simulink model "PE_V2_0"  (R2020b)
settings: Solver=VariableStepAuto  StartTime=0.0  StopTime=10.0  RelTol=1e-3
undefined symbols (not defined in the file): ZERO
libraries: hdlsllib x35, simulink x28, visionhdlutilities x12
(part 1 of 3)
settings Model: Creator=Xiao  LastModifiedBy=Xiao

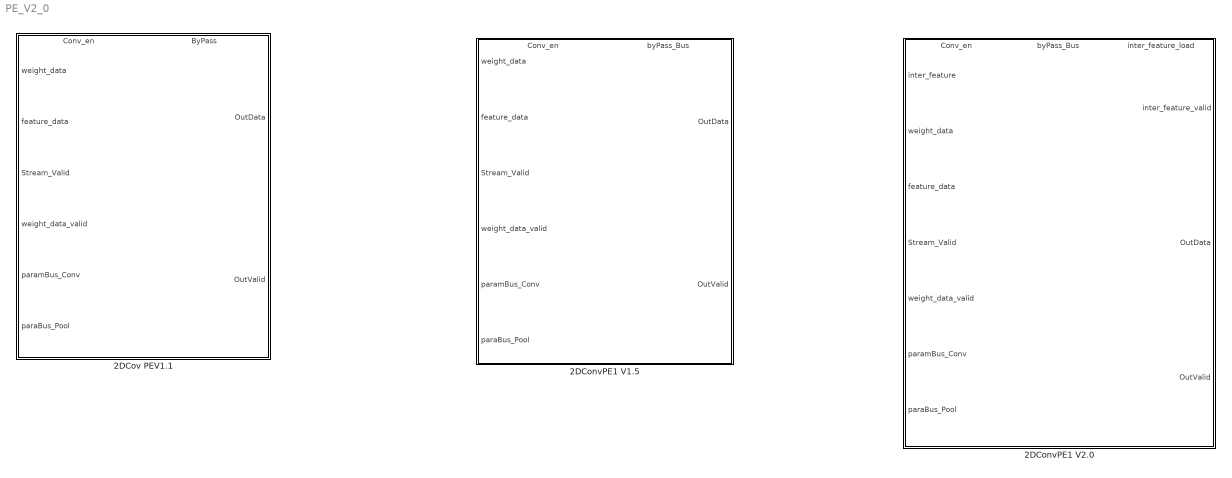
== system PE_V2_0 ==
  2DConvPE1 V1.5 : Subsystem
      settings: PortSchema="{\"entries\":[{\"content\":{\"sides\":[{\"content\":{\"connectorIds\":[\"In1\",\"In2\",\"In3\",\"In4\",\"In5\",\"In6\"]},\"type\":\"ConnectorPlacement.EquallySpacedRectSide\",\"uuid\":\"72a132f7-3e47-4ef1-8d79-baadbeb84817\"},{\"content\":{\"connectorIds\":[\"Out1\",\"Out2\"],\"side\":\"RIGHT\"},\"type\":\"ConnectorPlacement.EquallySpacedRectSide\",\"uuid\":\"2df9bf31-2175-4d97-aafa-a0227f37f2af\"},{\"content\":{\"connectorIds\":[\"In7\",\"In8\"],\"side\":\"TOP\"},\"type\":\"ConnectorPlacement.EquallySpacedRectSide\",\"uuid\":\"1b8495b8-ab7c-42d9-b044-413e20debbac\"},{\"content\":{\"connectorIds\":[],\"side\":\"BOTTOM\"},\"type\":\"ConnectorPlacement.EquallySpacedRectSide\",\"uuid\":\"e68361ac-7f7b-4816-948a-9cecfdd8f729\"},{\"content\":{\"connectorIds\":[],\"side\":\"HIDDEN\"},\"type\":\"ConnectorPlacement.EquallySpacedRectSide\",\"uuid\":\"818be012-dd2c-438f-8537-4d3d95a16bb4\"}]},\"type\":\"ConnectorPlacement.EquallySpacedConnector\",\"uuid\":\"cbadf64c-68f0-4765-b1bf-d60756169ff2\"}],\"packageUris\":[\"http://schema.mathworks.com/mf0/Connector/R2020b\"],\"version\":\"1.0\"}"
  2DConvPE1 V2.0 : Subsystem
      settings: PortSchema="{\"entries\":[{\"content\":{\"sides\":[{\"content\":{\"connectorIds\":[\"In1\",\"In2\",\"In3\",\"In4\",\"In5\",\"In6\",\"In7\"]},\"type\":\"ConnectorPlacement.EquallySpacedRectSide\",\"uuid\":\"72a132f7-3e47-4ef1-8d79-baadbeb84817\"},{\"content\":{\"connectorIds\":[\"Out1\",\"Out2\",\"Out3\"],\"side\":\"RIGHT\"},\"type\":\"ConnectorPlacement.EquallySpacedRectSide\",\"uuid\":\"2df9bf31-2175-4d97-aafa-a0227f37f2af\"},{\"content\":{\"connectorIds\":[\"In8\",\"In9\",\"In10\"],\"side\":\"TOP\"},\"type\":\"ConnectorPlacement.EquallySpacedRectSide\",\"uuid\":\"1b8495b8-ab7c-42d9-b044-413e20debbac\"},{\"content\":{\"connectorIds\":[],\"side\":\"BOTTOM\"},\"type\":\"ConnectorPlacement.EquallySpacedRectSide\",\"uuid\":\"e68361ac-7f7b-4816-948a-9cecfdd8f729\"},{\"content\":{\"connectorIds\":[],\"side\":\"HIDDEN\"},\"type\":\"ConnectorPlacement.EquallySpacedRectSide\",\"uuid\":\"818be012-dd2c-438f-8537-4d3d95a16bb4\"}]},\"type\":\"ConnectorPlacement.EquallySpacedConnector\",\"uuid\":\"cbadf64c-68f0-4765-b1bf-d60756169ff2\"}],\"packageUris\":[\"http://schema.mathworks.com/mf0/Connector/R2020b\"],\"version\":\"1.0\"}"
  2DCov PEV1.1 : Subsystem
      settings: PortSchema="{\"entries\":[{\"content\":{\"sides\":[{\"content\":{\"connectorIds\":[\"In1\",\"In2\",\"In3\",\"In4\",\"In5\",\"In6\"]},\"type\":\"ConnectorPlacement.EquallySpacedRectSide\",\"uuid\":\"72a132f7-3e47-4ef1-8d79-baadbeb84817\"},{\"content\":{\"connectorIds\":[\"Out1\",\"Out2\"],\"side\":\"RIGHT\"},\"type\":\"ConnectorPlacement.EquallySpacedRectSide\",\"uuid\":\"2df9bf31-2175-4d97-aafa-a0227f37f2af\"},{\"content\":{\"connectorIds\":[\"In7\",\"In8\"],\"side\":\"TOP\"},\"type\":\"ConnectorPlacement.EquallySpacedRectSide\",\"uuid\":\"1b8495b8-ab7c-42d9-b044-413e20debbac\"},{\"content\":{\"connectorIds\":[],\"side\":\"BOTTOM\"},\"type\":\"ConnectorPlacement.EquallySpacedRectSide\",\"uuid\":\"e68361ac-7f7b-4816-948a-9cecfdd8f729\"},{\"content\":{\"connectorIds\":[],\"side\":\"HIDDEN\"},\"type\":\"ConnectorPlacement.EquallySpacedRectSide\",\"uuid\":\"818be012-dd2c-438f-8537-4d3d95a16bb4\"}]},\"type\":\"ConnectorPlacement.EquallySpacedConnector\",\"uuid\":\"cbadf64c-68f0-4765-b1bf-d60756169ff2\"}],\"packageUris\":[\"http://schema.mathworks.com/mf0/Connector/R2020b\"],\"version\":\"1.0\"}"

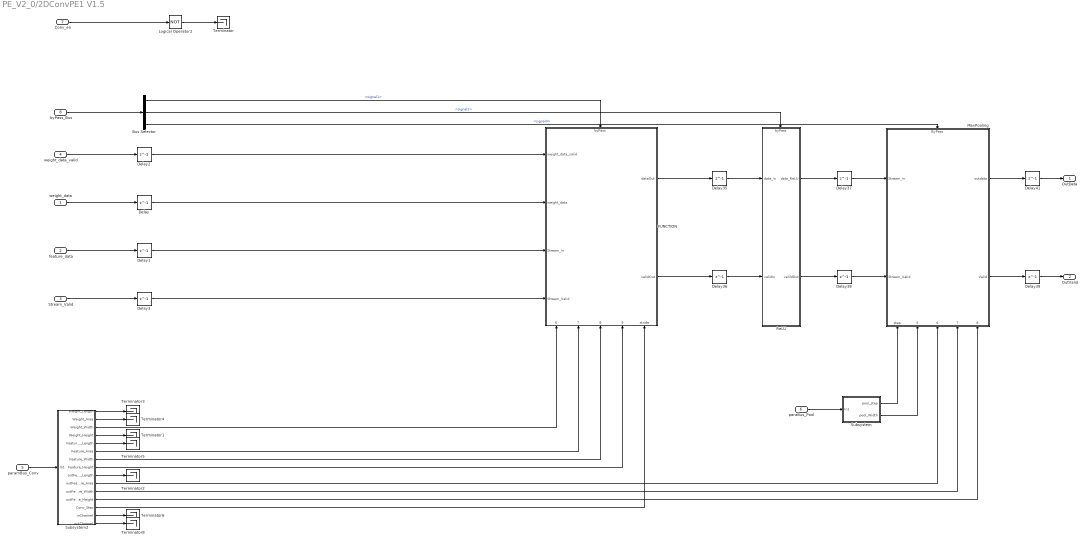
== system PE_V2_0/2DConvPE1 V1.5 ==
  weight_data : Inport
  feature_data : Inport  Port=2
  Stream_Valid : Inport  Port=3
  weight_data_valid : Inport  Port=4
  paramBus_Conv : Inport  Port=5
  paraBus_Pool : Inport  Port=6
  Conv_en : Inport  Port=7
  byPass_Bus : Inport  Port=8
  Bus Selector : BusSelector  OutputSignals=signal1,signal2,signal3
  Delay{,1..3,35..39,41} (10 alike) : Delay  DelayLength=1
  FUNCTION : Subsystem
      settings: PortSchema="{\"entries\":[{\"content\":{\"sides\":[{\"content\":{\"connectorIds\":[\"In1\",\"In2\",\"In3\",\"In4\"]},\"type\":\"ConnectorPlacement.EquallySpacedRectSide\",\"uuid\":\"bed083cc-10ce-4f46-a724-2c2c82e71793\"},{\"content\":{\"connectorIds\":[\"Out1\",\"Out2\"],\"side\":\"RIGHT\"},\"type\":\"ConnectorPlacement.EquallySpacedRectSide\",\"uuid\":\"c0d53dd0-88dc-4789-a28b-52aa625e6829\"},{\"content\":{\"connectorIds\":[\"In5\"],\"side\":\"TOP\"},\"type\":\"ConnectorPlacement.EquallySpacedRectSide\",\"uuid\":\"1fc99caf-d887-47fd-8f7a-576d1660cb35\"},{\"content\":{\"connectorIds\":[\"In6\",\"In7\",\"In8\",\"In9\",\"In10\"],\"side\":\"BOTTOM\"},\"type\":\"ConnectorPlacement.EquallySpacedRectSide\",\"uuid\":\"c33a9856-e25e-4d20-97d3-ef7dd12e1c8d\"},{\"content\":{\"connectorIds\":[],\"side\":\"HIDDEN\"},\"type\":\"ConnectorPlacement.EquallySpacedRectSide\",\"uuid\":\"c30f7557-1904-42a6-8652-95c43c5090df\"}]},\"type\":\"ConnectorPlacement.EquallySpacedConnector\",\"uuid\":\"8e0cb07a-0a7c-4542-b766-635afc6aa2db\"}],\"packageUris\":[\"http://schema.mathworks.com/mf0/Connector/R2020b\"],\"version\":\"1.0\"}"
  Logical Operator2 : Logic  Operator=NOT  AllPortsSameDT=off  OutDataTypeStr=boolean
  MaxPooling : Subsystem
      settings: PortSchema="{\"entries\":[{\"content\":{\"sides\":[{\"content\":{\"connectorIds\":[\"In1\",\"In2\"]},\"type\":\"ConnectorPlacement.EquallySpacedRectSide\",\"uuid\":\"8f082555-10a5-4426-9c6d-30ad9c9edc83\"},{\"content\":{\"connectorIds\":[\"Out1\",\"Out2\"],\"side\":\"RIGHT\"},\"type\":\"ConnectorPlacement.EquallySpacedRectSide\",\"uuid\":\"2f08e48d-98a7-49ef-9240-49e9a92f7835\"},{\"content\":{\"connectorIds\":[\"In3\"],\"side\":\"TOP\"},\"type\":\"ConnectorPlacement.EquallySpacedRectSide\",\"uuid\":\"9c785374-bdb9-47d6-a84c-95016a7dac24\"},{\"content\":{\"connectorIds\":[\"In4\",\"In5\",\"In6\",\"In7\",\"In8\"],\"side\":\"BOTTOM\"},\"type\":\"ConnectorPlacement.EquallySpacedRectSide\",\"uuid\":\"81220b33-16bc-4efc-91f7-9bf9738f949c\"},{\"content\":{\"connectorIds\":[],\"side\":\"HIDDEN\"},\"type\":\"ConnectorPlacement.EquallySpacedRectSide\",\"uuid\":\"99d22b10-fe8c-4c64-8a09-c433657226d7\"}]},\"type\":\"ConnectorPlacement.EquallySpacedConnector\",\"uuid\":\"f09d9050-86eb-4a30-82a2-eebdb84e68d3\"}],\"packageUris\":[\"http://schema.mathworks.com/mf0/Connector/R2020b\"],\"version\":\"1.0\"}"
  ReLU : Subsystem
      settings: PortSchema="{\"entries\":[{\"content\":{\"sides\":[{\"content\":{\"connectorIds\":[\"In1\",\"In2\"]},\"type\":\"ConnectorPlacement.EquallySpacedRectSide\",\"uuid\":\"abc19905-3b44-4985-b45b-942e5eaa1386\"},{\"content\":{\"connectorIds\":[\"Out1\",\"Out2\"],\"side\":\"RIGHT\"},\"type\":\"ConnectorPlacement.EquallySpacedRectSide\",\"uuid\":\"b0a86706-72e5-448b-9f1b-a0967f50aac9\"},{\"content\":{\"connectorIds\":[\"In3\"],\"side\":\"TOP\"},\"type\":\"ConnectorPlacement.EquallySpacedRectSide\",\"uuid\":\"df5d57b0-52e5-439f-8896-63a90ec5378c\"},{\"content\":{\"connectorIds\":[],\"side\":\"HIDDEN\"},\"type\":\"ConnectorPlacement.EquallySpacedRectSide\",\"uuid\":\"493b8843-365c-4ea1-b4d2-a52d72a7a785\"}]},\"type\":\"ConnectorPlacement.EquallySpacedConnector\",\"uuid\":\"755c5668-4a5f-4120-9a22-1155c417e52d\"}],\"packageUris\":[\"http://schema.mathworks.com/mf0/Connector/R2020b\"],\"version\":\"1.0\"}"
  Subsystem : Subsystem
  Subsystem2 : Subsystem
  Terminator{,1..6,8} (8 alike) : Terminator
  OutData : Outport
  OutValid : Outport  Port=2
  wires:
  Conv_en/1 -> Logical Operator2/1
  Logical Operator2/1 -> Terminator/1
  Delay35/1 -> ReLU/1(data_in)
  ReLU/1(data_ReLU) -> Delay37/1
  MaxPooling/1(outdata) -> Delay41/1
  MaxPooling/2(Valid) -> Delay39/1
  paraBus_Pool/1 -> Subsystem/1(In1)
  Subsystem/1(pool_step) -> MaxPooling/4(step)
  Subsystem/2(pool_Width) -> MaxPooling/5(Window_Width)
  Subsystem2/11(outFeature_Width) -> MaxPooling/7(Feature_Width)
  Subsystem2/10(outFeature_Area) -> MaxPooling/6(Feature_Area)
  Subsystem2/12(outFeature_Height) -> MaxPooling/8(Feature_Height)
  paramBus_Conv/1 -> Subsystem2/1(In1)
  Subsystem2/14(inChannel) -> Terminator6/1
  Subsystem2/4(Weight_Height) -> Terminator1/1
  Subsystem2/9(outFeature_Length) -> Terminator2/1
  Subsystem2/1(Weight_Length) -> Terminator3/1
  Subsystem2/2(Weight_Area) -> Terminator4/1
  Subsystem2/5(Feature_Length) -> Terminator5/1
  Subsystem2/15(outChannel) -> Terminator8/1
  ReLU/2(valildOut) -> Delay38/1
  weight_data/1 -> Delay/1
  weight_data_valid/1 -> Delay2/1
  feature_data/1 -> Delay1/1
  Stream_Valid/1 -> Delay3/1
  Delay36/1 -> ReLU/2(validIn)
  Delay37/1 -> MaxPooling/1(Stream_In)
  Delay38/1 -> MaxPooling/2(Stream_Valid)
  Delay41/1 -> OutData/1
  Delay39/1 -> OutValid/1
  byPass_Bus/1 -> Bus Selector/1
  Bus Selector/3 -> MaxPooling/3(ByPass)  "<signal3>"
  Bus Selector/2 -> ReLU/3(byPass)  "<signal2>"
  Delay2/1 -> FUNCTION/1(weight_data_valid)
  Delay/1 -> FUNCTION/2(weight_data)
  Delay1/1 -> FUNCTION/3(Stream_In)
  Delay3/1 -> FUNCTION/4(Stream_Valid)
  Subsystem2/3(Weight_Width) -> FUNCTION/6(Weight_Width)
  Subsystem2/6(Feature_Area) -> FUNCTION/7(Feature_Area)
  Subsystem2/7(Feature_Width) -> FUNCTION/8(Feature_Width)
  Subsystem2/8(Feature_Height) -> FUNCTION/9(Feature_Height)
  Subsystem2/13(Conv_Step) -> FUNCTION/10(stride)
  FUNCTION/1(dataOut) -> Delay35/1
  FUNCTION/2(validOut) -> Delay36/1
  Bus Selector/1 -> FUNCTION/5(byPass)  "<signal1>"

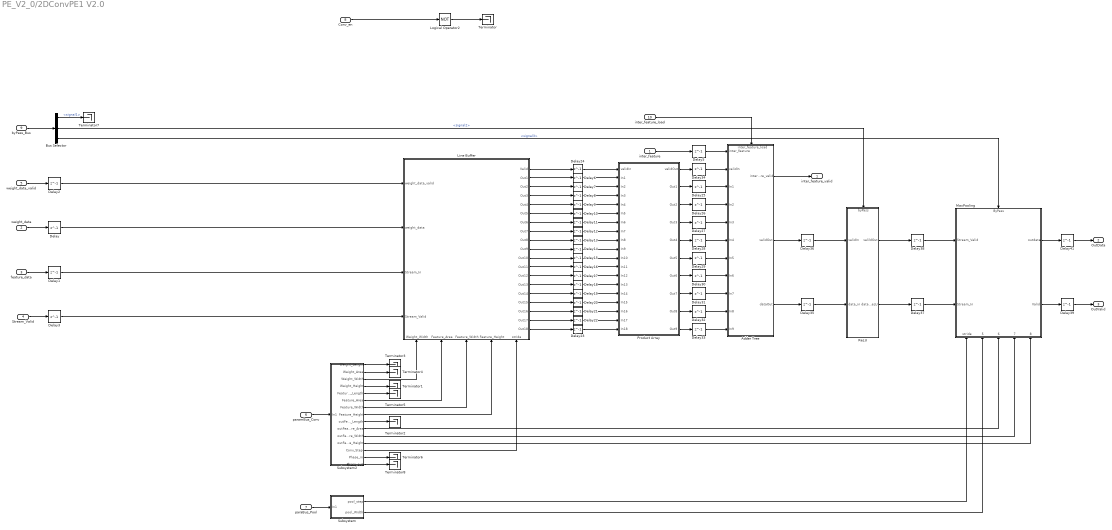
== system PE_V2_0/2DConvPE1 V2.0 ==
  inter_feature : Inport
  weight_data : Inport  Port=2
  feature_data : Inport  Port=3
  Stream_Valid : Inport  Port=4
  weight_data_valid : Inport  Port=5
  paramBus_Conv : Inport  Port=6
  paraBus_Pool : Inport  Port=7
  Conv_en : Inport  Port=8
  byPass_Bus : Inport  Port=9
  inter_feature_load : Inport  Port=10
  Adder Tree : Subsystem
      settings: PortSchema="{\"entries\":[{\"content\":{\"sides\":[{\"content\":{\"connectorIds\":[\"In1\",\"In2\",\"In3\",\"In4\",\"In5\",\"In6\",\"In7\",\"In8\",\"In9\",\"In10\",\"In11\"]},\"type\":\"ConnectorPlacement.EquallySpacedRectSide\",\"uuid\":\"a2770fc8-c2bb-4f97-8127-9a4f9dcf3825\"},{\"content\":{\"connectorIds\":[\"Out1\",\"Out2\",\"Out3\"],\"side\":\"RIGHT\"},\"type\":\"ConnectorPlacement.EquallySpacedRectSide\",\"uuid\":\"e7824c27-562b-441e-9955-8b5c243004da\"},{\"content\":{\"connectorIds\":[\"In12\"],\"side\":\"TOP\"},\"type\":\"ConnectorPlacement.EquallySpacedRectSide\",\"uuid\":\"ac1c8bec-6be4-4eb3-bc0e-7b7fb253fd27\"},{\"content\":{\"connectorIds\":[],\"side\":\"HIDDEN\"},\"type\":\"ConnectorPlacement.EquallySpacedRectSide\",\"uuid\":\"83260308-97e6-439f-9ad4-eb453db87a9c\"}]},\"type\":\"ConnectorPlacement.EquallySpacedConnector\",\"uuid\":\"e705b5d7-213e-4592-b0c5-9ab5c3365200\"}],\"packageUris\":[\"http://schema.mathworks.com/mf0/Connector/R2020b\"],\"version\":\"1.0\"}"
  Bus Selector : BusSelector  OutputSignals=signal1,signal2,signal3
  Delay{,1..3,5..39,41} (40 alike) : Delay  DelayLength=1
  Line Buffer : Subsystem
      settings: PortSchema="{\"entries\":[{\"content\":{\"sides\":[{\"content\":{\"connectorIds\":[\"In1\",\"In2\",\"In3\",\"In4\"]},\"type\":\"ConnectorPlacement.EquallySpacedRectSide\",\"uuid\":\"29b80ed8-848a-41c0-b6e7-f177bb4434f3\"},{\"content\":{\"connectorIds\":[\"Out1\",\"Out2\",\"Out3\",\"Out4\",\"Out5\",\"Out6\",\"Out7\",\"Out8\",\"Out9\",\"Out10\",\"Out11\",\"Out12\",\"Out13\",\"Out14\",\"Out15\",\"Out16\",\"Out17\",\"Out18\",\"Out19\"],\"side\":\"RIGHT\"},\"type\":\"ConnectorPlacement.EquallySpacedRectSide\",\"uuid\":\"adaf16a8-ce9f-43de-8b43-956a28d6fbef\"},{\"content\":{\"connectorIds\":[],\"side\":\"TOP\"},\"type\":\"ConnectorPlacement.EquallySpacedRectSide\",\"uuid\":\"106fd3d1-022d-44b8-9392-934ec241d21c\"},{\"content\":{\"connectorIds\":[\"In5\",\"In6\",\"In7\",\"In8\",\"In9\"],\"side\":\"BOTTOM\"},\"type\":\"ConnectorPlacement.EquallySpacedRectSide\",\"uuid\":\"8507e472-68b8-4fe5-bb7c-5a7beeecdd12\"},{\"content\":{\"connectorIds\":[],\"side\":\"HIDDEN\"},\"type\":\"ConnectorPlacement.EquallySpacedRectSide\",\"uuid\":\"f49b73e9-0f9f-4778-9ce1-2ad9bbb71891\"}]},\"type\":\"ConnectorPlacement.EquallySpacedConnector\",\"uuid\":\"21a60f11-360c-44f0-bdd6-bae5bf125dc3\"}],\"packageUris\":[\"http://schema.mathworks.com/mf0/Connector/R2020b\"],\"version\":\"1.0\"}"
  Logical Operator2 : Logic  Operator=NOT  AllPortsSameDT=off  OutDataTypeStr=boolean
  MaxPooling : Subsystem
      settings: PortSchema="{\"entries\":[{\"content\":{\"sides\":[{\"content\":{\"connectorIds\":[\"In1\",\"In2\"]},\"type\":\"ConnectorPlacement.EquallySpacedRectSide\",\"uuid\":\"8f082555-10a5-4426-9c6d-30ad9c9edc83\"},{\"content\":{\"connectorIds\":[\"Out1\",\"Out2\"],\"side\":\"RIGHT\"},\"type\":\"ConnectorPlacement.EquallySpacedRectSide\",\"uuid\":\"2f08e48d-98a7-49ef-9240-49e9a92f7835\"},{\"content\":{\"connectorIds\":[\"In3\"],\"side\":\"TOP\"},\"type\":\"ConnectorPlacement.EquallySpacedRectSide\",\"uuid\":\"9c785374-bdb9-47d6-a84c-95016a7dac24\"},{\"content\":{\"connectorIds\":[\"In4\",\"In5\",\"In6\",\"In7\",\"In8\"],\"side\":\"BOTTOM\"},\"type\":\"ConnectorPlacement.EquallySpacedRectSide\",\"uuid\":\"81220b33-16bc-4efc-91f7-9bf9738f949c\"},{\"content\":{\"connectorIds\":[],\"side\":\"HIDDEN\"},\"type\":\"ConnectorPlacement.EquallySpacedRectSide\",\"uuid\":\"99d22b10-fe8c-4c64-8a09-c433657226d7\"}]},\"type\":\"ConnectorPlacement.EquallySpacedConnector\",\"uuid\":\"f09d9050-86eb-4a30-82a2-eebdb84e68d3\"}],\"packageUris\":[\"http://schema.mathworks.com/mf0/Connector/R2020b\"],\"version\":\"1.0\"}"
  Product Array : Subsystem
  ReLU : Subsystem
      settings: PortSchema="{\"entries\":[{\"content\":{\"sides\":[{\"content\":{\"connectorIds\":[\"In1\",\"In2\"]},\"type\":\"ConnectorPlacement.EquallySpacedRectSide\",\"uuid\":\"abc19905-3b44-4985-b45b-942e5eaa1386\"},{\"content\":{\"connectorIds\":[\"Out1\",\"Out2\"],\"side\":\"RIGHT\"},\"type\":\"ConnectorPlacement.EquallySpacedRectSide\",\"uuid\":\"b0a86706-72e5-448b-9f1b-a0967f50aac9\"},{\"content\":{\"connectorIds\":[\"In3\"],\"side\":\"TOP\"},\"type\":\"ConnectorPlacement.EquallySpacedRectSide\",\"uuid\":\"df5d57b0-52e5-439f-8896-63a90ec5378c\"},{\"content\":{\"connectorIds\":[],\"side\":\"HIDDEN\"},\"type\":\"ConnectorPlacement.EquallySpacedRectSide\",\"uuid\":\"493b8843-365c-4ea1-b4d2-a52d72a7a785\"}]},\"type\":\"ConnectorPlacement.EquallySpacedConnector\",\"uuid\":\"755c5668-4a5f-4120-9a22-1155c417e52d\"}],\"packageUris\":[\"http://schema.mathworks.com/mf0/Connector/R2020b\"],\"version\":\"1.0\"}"
  Subsystem : Subsystem
  Subsystem2 : Subsystem
  Terminator{,1..8} (9 alike) : Terminator
  inter_feature_valid : Outport
  OutData : Outport  Port=2
  OutValid : Outport  Port=3
  wires:
  Conv_en/1 -> Logical Operator2/1
  Logical Operator2/1 -> Terminator/1
  Delay35/1 -> ReLU/2(data_in)
  ReLU/2(data_ReLU) -> Delay37/1
  MaxPooling/1(outdata) -> Delay41/1
  MaxPooling/2(Valid) -> Delay39/1
  paraBus_Pool/1 -> Subsystem/1(In1)
  Subsystem/1(pool_step) -> MaxPooling/4(stride)
  Subsystem/2(pool_Width) -> MaxPooling/5(Window_Width)
  Subsystem2/11(outFeature_Width) -> MaxPooling/7(Feature_Width)
  Subsystem2/10(outFeature_Area) -> MaxPooling/6(Feature_Area)
  Subsystem2/12(outFeature_Height) -> MaxPooling/8(Feature_Height)
  paramBus_Conv/1 -> Subsystem2/1(In1)
  Subsystem2/14(Phase_in) -> Terminator6/1
  Subsystem2/4(Weight_Height) -> Terminator1/1
  Subsystem2/9(outFeature_Length) -> Terminator2/1
  Subsystem2/1(Weight_Length) -> Terminator3/1
  Subsystem2/2(Weight_Area) -> Terminator4/1
  Subsystem2/5(Feature_Length) -> Terminator5/1
  Subsystem2/15(Phase_out) -> Terminator8/1
  ReLU/1(valildOut) -> Delay38/1
  weight_data/1 -> Delay/1
  weight_data_valid/1 -> Delay2/1
  feature_data/1 -> Delay1/1
  Stream_Valid/1 -> Delay3/1
  Delay36/1 -> ReLU/1(validIn)
  Delay37/1 -> MaxPooling/2(Stream_In)
  Delay38/1 -> MaxPooling/1(Stream_Valid)
  Delay41/1 -> OutData/1
  Delay39/1 -> OutValid/1
  byPass_Bus/1 -> Bus Selector/1
  Bus Selector/3 -> MaxPooling/3(ByPass)  "<signal3>"
  Bus Selector/2 -> ReLU/3(byPass)  "<signal2>"
  Adder Tree/3(dataOut) -> Delay35/1
  Adder Tree/2(validOut) -> Delay36/1
  Delay3/1 -> Line Buffer/4(Stream_Valid)
  Delay1/1 -> Line Buffer/3(Stream_In)
  Delay/1 -> Line Buffer/2(weight_data)
  Delay2/1 -> Line Buffer/1(weight_data_valid)
  Subsystem2/8(Feature_Height) -> Line Buffer/8(Feature_Height)
  Subsystem2/6(Feature_Area) -> Line Buffer/6(Feature_Area)
  Subsystem2/3(Weight_Width) -> Line Buffer/5(Weight_Width)
  Line Buffer/6(Out5) -> Delay10/1
  Line Buffer/5(Out4) -> Delay9/1
  Line Buffer/13(Out12) -> Delay17/1
  Line Buffer/3(Out2) -> Delay7/1
  Line Buffer/9(Out8) -> Delay13/1
  Line Buffer/8(Out7) -> Delay12/1
  Delay25/1 -> Adder Tree/3(In1)
  Line Buffer/7(Out6) -> Delay11/1
  Delay27/1 -> Adder Tree/5(In3)
  Delay29/1 -> Adder Tree/7(In5)
  Line Buffer/17(Out16) -> Delay21/1
  Delay26/1 -> Adder Tree/4(In2)
  Product Array/2(Out1) -> Delay25/1
  Delay33/1 -> Adder Tree/11(In9)
  Product Array/1(validOut) -> Delay34/1
  Product Array/9(Out8) -> Delay32/1
  Line Buffer/11(Out10) -> Delay15/1
  Delay30/1 -> Adder Tree/8(In6)
  Line Buffer/15(Out14) -> Delay19/1
  Delay31/1 -> Adder Tree/9(In7)
  Product Array/3(Out2) -> Delay26/1
  Product Array/5(Out4) -> Delay28/1
  Delay32/1 -> Adder Tree/10(In8)
  Product Array/6(Out5) -> Delay29/1
  Product Array/4(Out3) -> Delay27/1
  Line Buffer/4(Out3) -> Delay8/1
  Product Array/10(Out9) -> Delay33/1
  Delay24/1 -> Product Array/1(validIn)
  Delay28/1 -> Adder Tree/6(In4)
  Delay23/1 -> Product Array/19(In18)
  Subsystem2/13(Conv_Step) -> Line Buffer/9(stride)
  Product Array/8(Out7) -> Delay31/1
  Delay16/1 -> Product Array/12(In11)
  Delay19/1 -> Product Array/15(In14)
  Delay21/1 -> Product Array/17(In16)
  Delay17/1 -> Product Array/13(In12)
  Delay8/1 -> Product Array/4(In3)
  Line Buffer/12(Out11) -> Delay16/1
  Delay22/1 -> Product Array/18(In17)
  Delay14/1 -> Product Array/10(In9)
  Line Buffer/19(Out18) -> Delay23/1
  Line Buffer/2(Out1) -> Delay6/1
  Delay15/1 -> Product Array/11(In10)
  Line Buffer/16(Out15) -> Delay20/1
  Delay34/1 -> Adder Tree/2(validIn)
  Delay11/1 -> Product Array/7(In6)
  Line Buffer/18(Out17) -> Delay22/1
  Delay13/1 -> Product Array/9(In8)
  Line Buffer/14(Out13) -> Delay18/1
  Delay9/1 -> Product Array/5(In4)
  Delay20/1 -> Product Array/16(In15)
  Delay18/1 -> Product Array/14(In13)
  Subsystem2/7(Feature_Width) -> Line Buffer/7(Feature_Width)
  Delay12/1 -> Product Array/8(In7)
  Delay10/1 -> Product Array/6(In5)
  Delay6/1 -> Product Array/2(In1)
  Line Buffer/1(Valid) -> Delay24/1
  Product Array/7(Out6) -> Delay30/1
  Delay7/1 -> Product Array/3(In2)
  Line Buffer/10(Out9) -> Delay14/1
  Bus Selector/1 -> Terminator7/1  "<signal1>"
  inter_feature/1 -> Delay5/1
  Delay5/1 -> Adder Tree/1(inter_feature)
  inter_feature_load/1 -> Adder Tree/12(inter_feature_load)
  Adder Tree/1(inter_feature_valid) -> inter_feature_valid/1

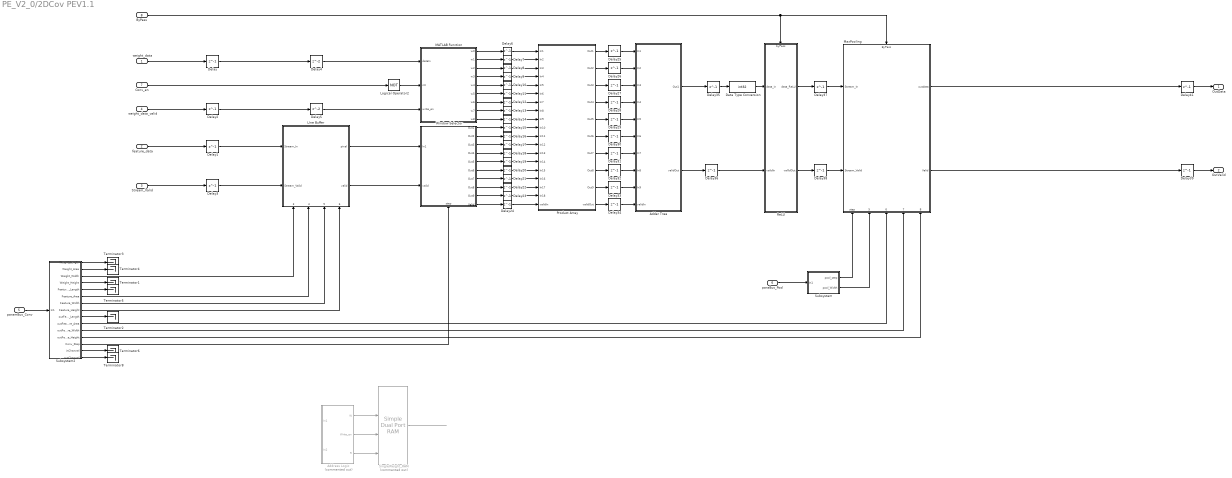
== system PE_V2_0/2DCov PEV1.1 ==
  weight_data : Inport
  feature_data : Inport  Port=2
  Stream_Valid : Inport  Port=3
  weight_data_valid : Inport  Port=4
  paramBus_Conv : Inport  Port=5
  paraBus_Pool : Inport  Port=6
  Conv_en : Inport  Port=7
  ByPass : Inport  Port=8
  Adder Tree : Subsystem
  Address Logic : Subsystem  Commented=on
  Data Type Conversion : DataTypeConversion  OutDataTypeStr=int32
  Delay{,1..3,6..39,41} (39 alike) : Delay  DelayLength=1
  Delay4 : Delay
  Delay5 : Delay
  LIne Buffer : Subsystem
      settings: PortSchema="{\"entries\":[{\"content\":{\"sides\":[{\"content\":{\"connectorIds\":[\"In1\",\"In2\"]},\"type\":\"ConnectorPlacement.EquallySpacedRectSide\",\"uuid\":\"a250c848-7a40-462c-bfcf-0ff48046d99d\"},{\"content\":{\"connectorIds\":[\"Out1\",\"Out2\"],\"side\":\"RIGHT\"},\"type\":\"ConnectorPlacement.EquallySpacedRectSide\",\"uuid\":\"81aecf2d-6bfb-4d40-80c7-cfb89c921406\"},{\"content\":{\"connectorIds\":[],\"side\":\"TOP\"},\"type\":\"ConnectorPlacement.EquallySpacedRectSide\",\"uuid\":\"288ccc7a-b219-4526-a408-3d8b1082f4b0\"},{\"content\":{\"connectorIds\":[\"In3\",\"In4\",\"In5\",\"In6\"],\"side\":\"BOTTOM\"},\"type\":\"ConnectorPlacement.EquallySpacedRectSide\",\"uuid\":\"5d9529f5-ee70-4412-83ca-b280a2219284\"},{\"content\":{\"connectorIds\":[],\"side\":\"HIDDEN\"},\"type\":\"ConnectorPlacement.EquallySpacedRectSide\",\"uuid\":\"3d06d450-49b0-49ba-a273-690d97c3e8e1\"}]},\"type\":\"ConnectorPlacement.EquallySpacedConnector\",\"uuid\":\"b82e05d1-4695-4e04-9663-17698b30471b\"}],\"packageUris\":[\"http://schema.mathworks.com/mf0/Connector/R2020b\"],\"version\":\"1.0\"}"
  Logical Operator2 : Logic  Operator=NOT  AllPortsSameDT=off  OutDataTypeStr=boolean
  MATLAB Function : MATLAB Function  TreatAsAtomicUnit=on
  MaxPooling : Subsystem
      settings: PortSchema="{\"entries\":[{\"content\":{\"sides\":[{\"content\":{\"connectorIds\":[\"In1\",\"In2\"]},\"type\":\"ConnectorPlacement.EquallySpacedRectSide\",\"uuid\":\"8f082555-10a5-4426-9c6d-30ad9c9edc83\"},{\"content\":{\"connectorIds\":[\"Out1\",\"Out2\"],\"side\":\"RIGHT\"},\"type\":\"ConnectorPlacement.EquallySpacedRectSide\",\"uuid\":\"2f08e48d-98a7-49ef-9240-49e9a92f7835\"},{\"content\":{\"connectorIds\":[\"In3\"],\"side\":\"TOP\"},\"type\":\"ConnectorPlacement.EquallySpacedRectSide\",\"uuid\":\"9c785374-bdb9-47d6-a84c-95016a7dac24\"},{\"content\":{\"connectorIds\":[\"In4\",\"In5\",\"In6\",\"In7\",\"In8\"],\"side\":\"BOTTOM\"},\"type\":\"ConnectorPlacement.EquallySpacedRectSide\",\"uuid\":\"81220b33-16bc-4efc-91f7-9bf9738f949c\"},{\"content\":{\"connectorIds\":[],\"side\":\"HIDDEN\"},\"type\":\"ConnectorPlacement.EquallySpacedRectSide\",\"uuid\":\"99d22b10-fe8c-4c64-8a09-c433657226d7\"}]},\"type\":\"ConnectorPlacement.EquallySpacedConnector\",\"uuid\":\"f09d9050-86eb-4a30-82a2-eebdb84e68d3\"}],\"packageUris\":[\"http://schema.mathworks.com/mf0/Connector/R2020b\"],\"version\":\"1.0\"}"
  Product Array : Subsystem
  ReLU : Subsystem
      settings: PortSchema="{\"entries\":[{\"content\":{\"sides\":[{\"content\":{\"connectorIds\":[\"In1\",\"In2\"]},\"type\":\"ConnectorPlacement.EquallySpacedRectSide\",\"uuid\":\"abc19905-3b44-4985-b45b-942e5eaa1386\"},{\"content\":{\"connectorIds\":[\"Out1\",\"Out2\"],\"side\":\"RIGHT\"},\"type\":\"ConnectorPlacement.EquallySpacedRectSide\",\"uuid\":\"b0a86706-72e5-448b-9f1b-a0967f50aac9\"},{\"content\":{\"connectorIds\":[\"In3\"],\"side\":\"TOP\"},\"type\":\"ConnectorPlacement.EquallySpacedRectSide\",\"uuid\":\"df5d57b0-52e5-439f-8896-63a90ec5378c\"},{\"content\":{\"connectorIds\":[],\"side\":\"HIDDEN\"},\"type\":\"ConnectorPlacement.EquallySpacedRectSide\",\"uuid\":\"493b8843-365c-4ea1-b4d2-a52d72a7a785\"}]},\"type\":\"ConnectorPlacement.EquallySpacedConnector\",\"uuid\":\"755c5668-4a5f-4120-9a22-1155c417e52d\"}],\"packageUris\":[\"http://schema.mathworks.com/mf0/Connector/R2020b\"],\"version\":\"1.0\"}"
  SingleWeight_RAM : hdlsllib/HDL RAMs/Simple Dual Port RAM  Commented=on  ram_size=13
      settings: SourceProductName=HDL Coder
  Subsystem : Subsystem
  Subsystem2 : Subsystem
  Terminator{1..6,8} (7 alike) : Terminator
  Window Selector : Subsystem
      settings: PortSchema="{\"entries\":[{\"content\":{\"sides\":[{\"content\":{\"connectorIds\":[\"In1\",\"In2\"]},\"type\":\"ConnectorPlacement.EquallySpacedRectSide\",\"uuid\":\"2f98ee57-d732-418e-86bd-7acbaf2524e0\"},{\"content\":{\"connectorIds\":[\"Out1\",\"Out2\",\"Out3\",\"Out4\",\"Out5\",\"Out6\",\"Out7\",\"Out8\",\"Out9\",\"Out10\"],\"side\":\"RIGHT\"},\"type\":\"ConnectorPlacement.EquallySpacedRectSide\",\"uuid\":\"287ad403-178f-48f1-9791-2ccad363e9c6\"},{\"content\":{\"connectorIds\":[],\"side\":\"TOP\"},\"type\":\"ConnectorPlacement.EquallySpacedRectSide\",\"uuid\":\"a860ecae-5cde-45ef-a487-fdb4fb7390aa\"},{\"content\":{\"connectorIds\":[\"In3\"],\"side\":\"BOTTOM\"},\"type\":\"ConnectorPlacement.EquallySpacedRectSide\",\"uuid\":\"925435f5-0fb8-4a67-9f76-fe99b5b92634\"},{\"content\":{\"connectorIds\":[],\"side\":\"HIDDEN\"},\"type\":\"ConnectorPlacement.EquallySpacedRectSide\",\"uuid\":\"e6f3edac-a41a-4276-8ae6-cd8be9b02af9\"}]},\"type\":\"ConnectorPlacement.EquallySpacedConnector\",\"uuid\":\"0e32a9d0-da82-46c8-ab50-9de41c4380a9\"}],\"packageUris\":[\"http://schema.mathworks.com/mf0/Connector/R2020b\"],\"version\":\"1.0\"}"
  OutData : Outport
  OutValid : Outport  Port=2
  wires:
  Delay/1 -> Delay4/1
  Address Logic/1(W) -> SingleWeight_RAM/2
  Address Logic/2(Write_en) -> SingleWeight_RAM/3
  Address Logic/3(R) -> SingleWeight_RAM/4
  SingleWeight_RAM/1 -> ?
  Conv_en/1 -> Logical Operator2/1
  Delay2/1 -> Delay5/1
  Logical Operator2/1 -> MATLAB Function/2(rst)
  Adder Tree/1(Out1) -> Delay35/1
  Data Type Conversion/1 -> ReLU/1(data_in)
  ReLU/1(data_ReLU) -> Delay37/1
  ByPass/1 -> MaxPooling/3(ByPass), ReLU/3(byPass)
  MaxPooling/1(outdata) -> Delay41/1
  MaxPooling/2(Valid) -> Delay39/1
  paraBus_Pool/1 -> Subsystem/1(In1)
  Subsystem/1(pool_step) -> MaxPooling/4(step)
  Subsystem/2(pool_Width) -> MaxPooling/5(Window_Width)
  Subsystem2/11(outFeature_Width) -> MaxPooling/7(Feature_Width)
  Subsystem2/10(outFeature_Area) -> MaxPooling/6(Feature_Area)
  Subsystem2/12(outFeature_Height) -> MaxPooling/8(Feature_Height)
  paramBus_Conv/1 -> Subsystem2/1(In1)
  Subsystem2/14(inChannel) -> Terminator6/1
  Subsystem2/4(Weight_Height) -> Terminator1/1
  Subsystem2/9(outFeature_Length) -> Terminator2/1
  Subsystem2/13(Conv_Step) -> Window Selector/3(step)
  Subsystem2/1(Weight_Length) -> Terminator3/1
  Subsystem2/2(Weight_Area) -> Terminator4/1
  Subsystem2/5(Feature_Length) -> Terminator5/1
  Subsystem2/15(outChannel) -> Terminator8/1
  Adder Tree/2(validOut) -> Delay36/1
  ReLU/2(valildOut) -> Delay38/1
  Delay1/1 -> LIne Buffer/1(Stream_In)
  Delay3/1 -> LIne Buffer/2(Stream_Valid)
  Subsystem2/3(Weight_Width) -> LIne Buffer/3(Weight_Width)
  Subsystem2/6(Feature_Area) -> LIne Buffer/4(Feature_Area)
  Subsystem2/7(Feature_Width) -> LIne Buffer/5(Feature_Width)
  Subsystem2/8(Feature_Height) -> LIne Buffer/6(Feature_Height)
  LIne Buffer/1(pixel) -> Window Selector/1(In1)
  LIne Buffer/2(valid) -> Window Selector/2(valid)
  weight_data/1 -> Delay/1
  weight_data_valid/1 -> Delay2/1
  feature_data/1 -> Delay1/1
  Stream_Valid/1 -> Delay3/1
  Delay5/1 -> MATLAB Function/3(write_en)
  Delay4/1 -> MATLAB Function/1(dataIn)
  MATLAB Function/1(w0) -> Delay6/1
  Delay6/1 -> Product Array/1(In1)
  MATLAB Function/2(w1) -> Delay7/1
  Delay7/1 -> Product Array/2(In2)
  MATLAB Function/3(w2) -> Delay8/1
  Delay8/1 -> Product Array/3(In3)
  MATLAB Function/4(w3) -> Delay9/1
  Delay9/1 -> Product Array/4(In4)
  MATLAB Function/5(w4) -> Delay10/1
  Delay10/1 -> Product Array/5(In5)
  MATLAB Function/6(w5) -> Delay11/1
  Delay11/1 -> Product Array/6(In6)
  MATLAB Function/7(w6) -> Delay12/1
  Delay12/1 -> Product Array/7(In7)
  MATLAB Function/8(w7) -> Delay13/1
  Delay13/1 -> Product Array/8(In8)
  MATLAB Function/9(w8) -> Delay14/1
  Delay14/1 -> Product Array/9(In9)
  Window Selector/1(Out1) -> Delay15/1
  Delay15/1 -> Product Array/10(In10)
  Window Selector/2(Out2) -> Delay16/1
  Delay16/1 -> Product Array/11(In11)
  Window Selector/3(Out3) -> Delay17/1
  Delay17/1 -> Product Array/12(In12)
  Window Selector/4(Out4) -> Delay18/1
  Delay18/1 -> Product Array/13(In13)
  Window Selector/5(Out5) -> Delay19/1
  Delay19/1 -> Product Array/14(In14)
  Window Selector/6(Out6) -> Delay20/1
  Delay20/1 -> Product Array/15(In15)
  Window Selector/7(Out7) -> Delay21/1
  Delay21/1 -> Product Array/16(In16)
  Window Selector/8(Out8) -> Delay22/1
  Delay22/1 -> Product Array/17(In17)
  Window Selector/9(Out9) -> Delay23/1
  Delay23/1 -> Product Array/18(In18)
  Window Selector/10(Valid) -> Delay24/1
  Delay24/1 -> Product Array/19(validIn)
  Product Array/1(Out1) -> Delay25/1
  Delay25/1 -> Adder Tree/1(In1)
  Product Array/2(Out2) -> Delay26/1
  Product Array/3(Out3) -> Delay27/1
  Product Array/4(Out4) -> Delay28/1
  Product Array/5(Out5) -> Delay29/1
  Product Array/6(Out6) -> Delay30/1
  Product Array/7(Out7) -> Delay31/1
  Product Array/9(Out9) -> Delay33/1
  Product Array/8(Out8) -> Delay32/1
  Product Array/10(validOut) -> Delay34/1
  Delay26/1 -> Adder Tree/2(In2)
  Delay27/1 -> Adder Tree/3(In3)
  Delay28/1 -> Adder Tree/4(In4)
  Delay29/1 -> Adder Tree/5(In5)
  Delay30/1 -> Adder Tree/6(In6)
  Delay31/1 -> Adder Tree/7(In7)
  Delay32/1 -> Adder Tree/8(In8)
  Delay33/1 -> Adder Tree/9(In9)
  Delay34/1 -> Adder Tree/10(validIn)
  Delay35/1 -> Data Type Conversion/1
  Delay36/1 -> ReLU/2(validIn)
  Delay37/1 -> MaxPooling/1(Stream_In)
  Delay38/1 -> MaxPooling/2(Stream_Valid)
  Delay41/1 -> OutData/1
  Delay39/1 -> OutValid/1

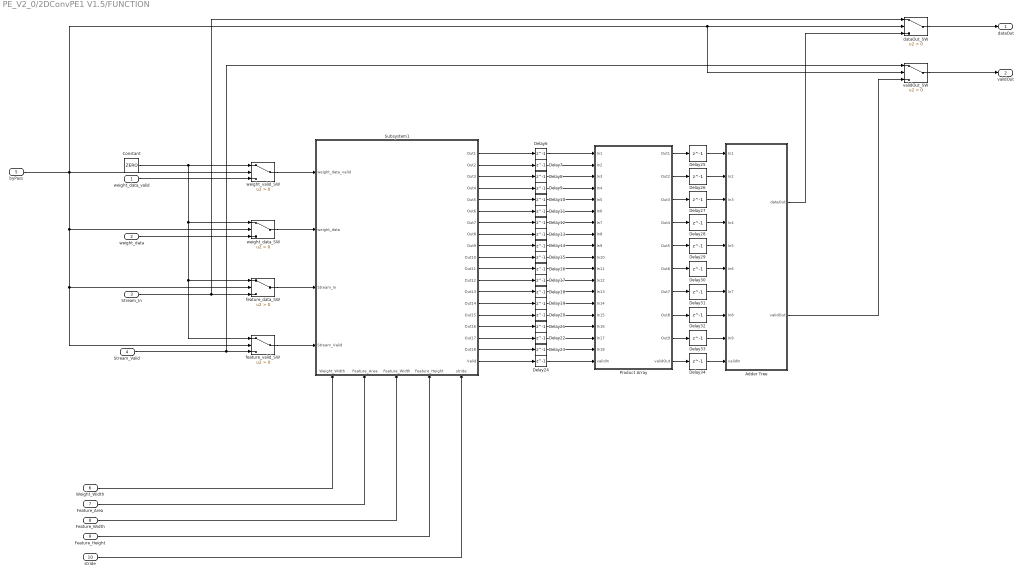
== system PE_V2_0/2DConvPE1 V1.5/FUNCTION ==
  weight_data_valid : Inport
  weight_data : Inport  Port=2
  Stream_In : Inport  Port=3
  Stream_Valid : Inport  Port=4
  byPass : Inport  Port=5
  Weight_Width : Inport  Port=6
  Feature_Area : Inport  Port=7
  Feature_Width : Inport  Port=8
  Feature_Height : Inport  Port=9
  stride : Inport  Port=10
  Adder Tree : Subsystem
  Constant : Constant  Value=ZERO
  Delay{6..34} (29 alike) : Delay  DelayLength=1
  Product Array : Subsystem
  Subsystem1 : Subsystem
      settings: PortSchema="{\"entries\":[{\"content\":{\"sides\":[{\"content\":{\"connectorIds\":[\"In1\",\"In2\",\"In3\",\"In4\"]},\"type\":\"ConnectorPlacement.EquallySpacedRectSide\",\"uuid\":\"29b80ed8-848a-41c0-b6e7-f177bb4434f3\"},{\"content\":{\"connectorIds\":[\"Out1\",\"Out2\",\"Out3\",\"Out4\",\"Out5\",\"Out6\",\"Out7\",\"Out8\",\"Out9\",\"Out10\",\"Out11\",\"Out12\",\"Out13\",\"Out14\",\"Out15\",\"Out16\",\"Out17\",\"Out18\",\"Out19\"],\"side\":\"RIGHT\"},\"type\":\"ConnectorPlacement.EquallySpacedRectSide\",\"uuid\":\"adaf16a8-ce9f-43de-8b43-956a28d6fbef\"},{\"content\":{\"connectorIds\":[],\"side\":\"TOP\"},\"type\":\"ConnectorPlacement.EquallySpacedRectSide\",\"uuid\":\"106fd3d1-022d-44b8-9392-934ec241d21c\"},{\"content\":{\"connectorIds\":[\"In5\",\"In6\",\"In7\",\"In8\",\"In9\"],\"side\":\"BOTTOM\"},\"type\":\"ConnectorPlacement.EquallySpacedRectSide\",\"uuid\":\"8507e472-68b8-4fe5-bb7c-5a7beeecdd12\"},{\"content\":{\"connectorIds\":[],\"side\":\"HIDDEN\"},\"type\":\"ConnectorPlacement.EquallySpacedRectSide\",\"uuid\":\"f49b73e9-0f9f-4778-9ce1-2ad9bbb71891\"}]},\"type\":\"ConnectorPlacement.EquallySpacedConnector\",\"uuid\":\"21a60f11-360c-44f0-bdd6-bae5bf125dc3\"}],\"packageUris\":[\"http://schema.mathworks.com/mf0/Connector/R2020b\"],\"version\":\"1.0\"}"
  dataOut_SW : Switch  Criteria=u2 > Threshold
  feature_data_SW : Switch  Criteria=u2 > Threshold
  feature_valid_SW : Switch  Criteria=u2 > Threshold
  validOut_SW : Switch  Criteria=u2 > Threshold
  weight_data_SW : Switch  Criteria=u2 > Threshold
  weight_valid_SW : Switch  Criteria=u2 > Threshold
  dataOut : Outport
  validOut : Outport  Port=2
  wires:
  Subsystem1/9(Out9) -> Delay14/1
  Delay7/1 -> Product Array/2(In2)
  Product Array/6(Out6) -> Delay30/1
  Subsystem1/19(Valid) -> Delay24/1
  Delay6/1 -> Product Array/1(In1)
  Delay10/1 -> Product Array/5(In5)
  Delay12/1 -> Product Array/7(In7)
  Feature_Width/1 -> Subsystem1/7(Feature_Width)
  weight_data/1 -> weight_data_SW/3
  Delay18/1 -> Product Array/13(In13)
  Delay20/1 -> Product Array/15(In15)
  Stream_In/1 -> dataOut_SW/1, feature_data_SW/3
  Delay9/1 -> Product Array/4(In4)
  Subsystem1/13(Out13) -> Delay18/1
  Delay13/1 -> Product Array/8(In8)
  Subsystem1/17(Out17) -> Delay22/1
  Delay11/1 -> Product Array/6(In6)
  Delay34/1 -> Adder Tree/10(validIn)
  Stream_Valid/1 -> validOut_SW/1, feature_valid_SW/3
  Subsystem1/15(Out15) -> Delay20/1
  Delay15/1 -> Product Array/10(In10)
  Subsystem1/1(Out1) -> Delay6/1
  Subsystem1/18(Out18) -> Delay23/1
  Delay14/1 -> Product Array/9(In9)
  weight_data_valid/1 -> weight_valid_SW/3
  Delay22/1 -> Product Array/17(In17)
  Adder Tree/1(dataOut) -> dataOut_SW/3
  Subsystem1/11(Out11) -> Delay16/1
  Delay8/1 -> Product Array/3(In3)
  Delay17/1 -> Product Array/12(In12)
  Delay21/1 -> Product Array/16(In16)
  Delay19/1 -> Product Array/14(In14)
  Delay16/1 -> Product Array/11(In11)
  Product Array/7(Out7) -> Delay31/1
  stride/1 -> Subsystem1/9(stride)
  Delay23/1 -> Product Array/18(In18)
  Adder Tree/2(validOut) -> validOut_SW/3
  Delay28/1 -> Adder Tree/4(In4)
  Delay24/1 -> Product Array/19(validIn)
  Product Array/9(Out9) -> Delay33/1
  Subsystem1/3(Out3) -> Delay8/1
  Product Array/3(Out3) -> Delay27/1
  Product Array/5(Out5) -> Delay29/1
  Delay32/1 -> Adder Tree/8(In8)
  Product Array/4(Out4) -> Delay28/1
  Product Array/2(Out2) -> Delay26/1
  Delay31/1 -> Adder Tree/7(In7)
  Subsystem1/14(Out14) -> Delay19/1
  Delay30/1 -> Adder Tree/6(In6)
  Subsystem1/10(Out10) -> Delay15/1
  Product Array/8(Out8) -> Delay32/1
  Product Array/10(validOut) -> Delay34/1
  Delay33/1 -> Adder Tree/9(In9)
  Product Array/1(Out1) -> Delay25/1
  Delay26/1 -> Adder Tree/2(In2)
  Subsystem1/16(Out16) -> Delay21/1
  Delay29/1 -> Adder Tree/5(In5)
  Delay27/1 -> Adder Tree/3(In3)
  Subsystem1/6(Out6) -> Delay11/1
  Delay25/1 -> Adder Tree/1(In1)
  Subsystem1/7(Out7) -> Delay12/1
  Subsystem1/8(Out8) -> Delay13/1
  Subsystem1/2(Out2) -> Delay7/1
  Subsystem1/12(Out12) -> Delay17/1
  Subsystem1/4(Out4) -> Delay9/1
  Subsystem1/5(Out5) -> Delay10/1
  Weight_Width/1 -> Subsystem1/5(Weight_Width)
  Feature_Area/1 -> Subsystem1/6(Feature_Area)
  Feature_Height/1 -> Subsystem1/8(Feature_Height)
  byPass/1 -> validOut_SW/2, dataOut_SW/2, weight_valid_SW/2, feature_valid_SW/2, feature_data_SW/2, weight_data_SW/2
  Constant/1 -> feature_valid_SW/1, feature_data_SW/1, weight_data_SW/1, weight_valid_SW/1
  weight_valid_SW/1 -> Subsystem1/1(weight_data_valid)
  weight_data_SW/1 -> Subsystem1/2(weight_data)
  feature_data_SW/1 -> Subsystem1/3(Stream_In)
  feature_valid_SW/1 -> Subsystem1/4(Stream_Valid)
  validOut_SW/1 -> validOut/1
  dataOut_SW/1 -> dataOut/1

== system PE_V2_0/2DConvPE1 V1.5/MaxPooling ==
  Stream_In : Inport
  Stream_Valid : Inport  Port=2
  ByPass : Inport  Port=3
  step : Inport  Port=4
  Window_Width : Inport  Port=5
  Feature_Area : Inport  Port=6
  Feature_Width : Inport  Port=7
  Feature_Height : Inport  Port=8
  Comparator : Subsystem
  Constant : Constant  Value=0  OutDataTypeStr=int32
  Delay{,1..6,36} (8 alike) : Delay  DelayLength=1
  Line Buffer1 : Subsystem
  OutValidGen : Subsystem
  Switch : Switch  Criteria=u2 > Threshold
  Switch1 : Switch  Criteria=u2 > Threshold
  Terminator1 : Terminator
  dataSwitch : Switch  Criteria=u2 > Threshold
  validSwitch : Switch  Criteria=u2 > Threshold
  window Selector : Subsystem
  outdata : Outport
  Valid : Outport  Port=2
  wires:
  window Selector/3(Out3) -> Delay3/1
  OutValidGen/1(Out1) -> window Selector/2(valid)
  Feature_Width/1 -> Line Buffer1/4(Feature_Width)
  Line Buffer1/3(shftEnable) -> Terminator1/1
  Window_Width/1 -> OutValidGen/2(Window_Width)
  window Selector/5(Valid) -> Delay5/1
  window Selector/1(Out1) -> Delay/1
  Line Buffer1/1(pixel) -> Delay2/1
  Line Buffer1/2(ctrl) -> OutValidGen/1(ctrl)
  window Selector/2(Out2) -> Delay6/1
  window Selector/4(Out4) -> Delay4/1
  Feature_Area/1 -> Line Buffer1/3(Feature_Area)
  Feature_Height/1 -> OutValidGen/3(Feature_Height)
  step/1 -> window Selector/3(step)
  Delay1/1 -> validSwitch/1, Switch1/3
  Comparator/1(Out1) -> dataSwitch/3
  Delay36/1 -> dataSwitch/1, Switch/3
  ByPass/1 -> validSwitch/2, dataSwitch/2, Switch1/2, Switch/2
  dataSwitch/1 -> outdata/1
  validSwitch/1 -> Valid/1
  Constant/1 -> Switch1/1, Switch/1
  Switch/1 -> Line Buffer1/1(Stream_In)
  Switch1/1 -> Line Buffer1/2(Stream_Valid)
  Comparator/2(outvalid) -> validSwitch/3
  Stream_In/1 -> Delay36/1
  Stream_Valid/1 -> Delay1/1
  Delay2/1 -> window Selector/1(pixel)
  Delay/1 -> Comparator/1(In1)
  Delay5/1 -> Comparator/5(Valid)
  Delay4/1 -> Comparator/4(In4)
  Delay3/1 -> Comparator/3(In3)
  Delay6/1 -> Comparator/2(In2)

== system PE_V2_0/2DConvPE1 V1.5/ReLU ==
  data_in : Inport
  validIn : Inport  Port=2
  byPass : Inport  Port=3
  Compare To Zero : simulink/Logic and Bit Operations/Compare To Zero  relop=>  OutDataTypeStr=boolean
  Constant : Constant  Value=0  OutDataTypeStr=int32
  Delay1 : Delay  DelayLength=1
  Delay36 : Delay  DelayLength=1
  Switch : Switch  Criteria=u2 > Threshold
  Switch1 : Switch  Criteria=u2 > Threshold
  data_ReLU : Outport
  valildOut : Outport  Port=2
  wires:
  Constant/1 -> Switch/3
  Delay36/1 -> Switch1/1, Switch/1, Compare To Zero/1
  Compare To Zero/1 -> Switch/2
  Switch/1 -> Switch1/3
  byPass/1 -> Switch1/2
  Switch1/1 -> data_ReLU/1
  Delay1/1 -> valildOut/1
  data_in/1 -> Delay36/1
  validIn/1 -> Delay1/1

== system PE_V2_0/2DConvPE1 V1.5/Subsystem ==
  In1 : Inport
  Bus Selector : BusSelector  OutputSignals=signal1,signal2
  pool_step : Outport
  pool_Width : Outport  Port=2
  wires:
  Bus Selector/2 -> pool_Width/1  "<signal2>"
  Bus Selector/1 -> pool_step/1  "<signal1>"
  In1/1 -> Bus Selector/1

== system PE_V2_0/2DConvPE1 V1.5/Subsystem2 ==
  In1 : Inport
  Bus Selector : BusSelector  OutputSignals=signal1,signal2,signal3,signal4,signal5,signal6,signal7,signal8,signal9,signal10,signal11,signal12,signal13,signal14,signal15
  Weight_Length : Outport
  Weight_Area : Outport  Port=2
  Weight_Width : Outport  Port=3
  Weight_Height : Outport  Port=4
  Feature_Length : Outport  Port=5
  Feature_Area : Outport  Port=6
  Feature_Width : Outport  Port=7
  Feature_Height : Outport  Port=8
  outFeature_Length : Outport  Port=9
  outFeature_Area : Outport  Port=10
  outFeature_Width : Outport  Port=11
  outFeature_Height : Outport  Port=12
  Conv_Step : Outport  Port=13
  inChannel : Outport  Port=14
  outChannel : Outport  Port=15
  wires:
  In1/1 -> Bus Selector/1
  Bus Selector/1 -> Weight_Length/1  "<signal1>"
  Bus Selector/2 -> Weight_Area/1  "<signal2>"
  Bus Selector/3 -> Weight_Width/1  "<signal3>"
  Bus Selector/4 -> Weight_Height/1  "<signal4>"
  Bus Selector/5 -> Feature_Length/1  "<signal5>"
  Bus Selector/6 -> Feature_Area/1  "<signal6>"
  Bus Selector/7 -> Feature_Width/1  "<signal7>"
  Bus Selector/8 -> Feature_Height/1  "<signal8>"
  Bus Selector/9 -> outFeature_Length/1  "<signal9>"
  Bus Selector/10 -> outFeature_Area/1  "<signal10>"
  Bus Selector/11 -> outFeature_Width/1  "<signal11>"
  Bus Selector/12 -> outFeature_Height/1  "<signal12>"
  Bus Selector/13 -> Conv_Step/1  "<signal13>"
  Bus Selector/14 -> inChannel/1  "<signal14>"
  Bus Selector/15 -> outChannel/1  "<signal15>"

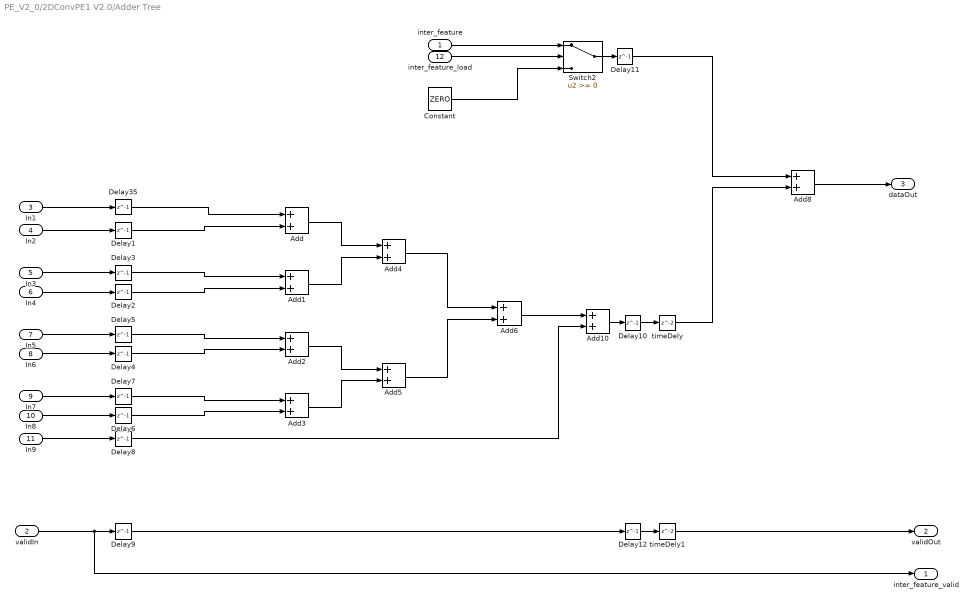
== system PE_V2_0/2DConvPE1 V2.0/Adder Tree ==
  inter_feature : Inport
  validIn : Inport  Port=2
  In1 : Inport  Port=3
  In2 : Inport  Port=4
  In3 : Inport  Port=5
  In4 : Inport  Port=6
  In5 : Inport  Port=7
  In6 : Inport  Port=8
  In7 : Inport  Port=9
  In8 : Inport  Port=10
  In9 : Inport  Port=11
  inter_feature_load : Inport  Port=12
  Add{,1..6,8,10} (9 alike) : Sum
  Constant : Constant  Value=ZERO  SampleTime=-1
  Delay{1..12,35} (13 alike) : Delay  DelayLength=1
  Switch2 : Switch
  timeDely : Delay
  timeDely1 : Delay
  inter_feature_valid : Outport
  validOut : Outport  Port=2
  dataOut : Outport  Port=3
  wires:
  Add/1 -> Add4/1
  Add4/1 -> Add6/1
  Add10/1 -> Delay10/1
  Add3/1 -> Add5/2
  Add2/1 -> Add5/1
  Add1/1 -> Add4/2
  Add6/1 -> Add10/1
  Add5/1 -> Add6/2
  Delay35/1 -> Add/1
  Delay1/1 -> Add/2
  Delay3/1 -> Add1/1
  Delay2/1 -> Add1/2
  Delay5/1 -> Add2/1
  Delay4/1 -> Add2/2
  Delay7/1 -> Add3/1
  Delay6/1 -> Add3/2
  In9/1 -> Delay8/1
  Delay8/1 -> Add10/2
  In8/1 -> Delay6/1
  In7/1 -> Delay7/1
  In6/1 -> Delay4/1
  In5/1 -> Delay5/1
  In4/1 -> Delay2/1
  In3/1 -> Delay3/1
  In2/1 -> Delay1/1
  In1/1 -> Delay35/1
  Delay9/1 -> Delay12/1
  inter_feature/1 -> Switch2/1
  validIn/1 -> inter_feature_valid/1, Delay9/1
  inter_feature_load/1 -> Switch2/2
  Constant/1 -> Switch2/3
  Switch2/1 -> Delay11/1
  Delay11/1 -> Add8/1
  Add8/1 -> dataOut/1
  Delay10/1 -> timeDely/1
  Delay12/1 -> timeDely1/1
  timeDely/1 -> Add8/2
  timeDely1/1 -> validOut/1

== system PE_V2_0/2DConvPE1 V2.0/Line Buffer ==
  weight_data_valid : Inport
  weight_data : Inport  Port=2
  Stream_In : Inport  Port=3
  Stream_Valid : Inport  Port=4
  Weight_Width : Inport  Port=5
  Feature_Area : Inport  Port=6
  Feature_Width : Inport  Port=7
  Feature_Height : Inport  Port=8
  stride : Inport  Port=9
  Delay4 : Delay
  Delay5 : Delay
  LIne Buffer : Subsystem
      settings: PortSchema="{\"entries\":[{\"content\":{\"sides\":[{\"content\":{\"connectorIds\":[\"In1\",\"In2\"]},\"type\":\"ConnectorPlacement.EquallySpacedRectSide\",\"uuid\":\"a250c848-7a40-462c-bfcf-0ff48046d99d\"},{\"content\":{\"connectorIds\":[\"Out1\",\"Out2\"],\"side\":\"RIGHT\"},\"type\":\"ConnectorPlacement.EquallySpacedRectSide\",\"uuid\":\"81aecf2d-6bfb-4d40-80c7-cfb89c921406\"},{\"content\":{\"connectorIds\":[],\"side\":\"TOP\"},\"type\":\"ConnectorPlacement.EquallySpacedRectSide\",\"uuid\":\"288ccc7a-b219-4526-a408-3d8b1082f4b0\"},{\"content\":{\"connectorIds\":[\"In3\",\"In4\",\"In5\",\"In6\"],\"side\":\"BOTTOM\"},\"type\":\"ConnectorPlacement.EquallySpacedRectSide\",\"uuid\":\"5d9529f5-ee70-4412-83ca-b280a2219284\"},{\"content\":{\"connectorIds\":[],\"side\":\"HIDDEN\"},\"type\":\"ConnectorPlacement.EquallySpacedRectSide\",\"uuid\":\"3d06d450-49b0-49ba-a273-690d97c3e8e1\"}]},\"type\":\"ConnectorPlacement.EquallySpacedConnector\",\"uuid\":\"b82e05d1-4695-4e04-9663-17698b30471b\"}],\"packageUris\":[\"http://schema.mathworks.com/mf0/Connector/R2020b\"],\"version\":\"1.0\"}"
  Window Selector : Subsystem
      settings: PortSchema="{\"entries\":[{\"content\":{\"sides\":[{\"content\":{\"connectorIds\":[\"In1\",\"In2\"]},\"type\":\"ConnectorPlacement.EquallySpacedRectSide\",\"uuid\":\"2f98ee57-d732-418e-86bd-7acbaf2524e0\"},{\"content\":{\"connectorIds\":[\"Out1\",\"Out2\",\"Out3\",\"Out4\",\"Out5\",\"Out6\",\"Out7\",\"Out8\",\"Out9\",\"Out10\"],\"side\":\"RIGHT\"},\"type\":\"ConnectorPlacement.EquallySpacedRectSide\",\"uuid\":\"287ad403-178f-48f1-9791-2ccad363e9c6\"},{\"content\":{\"connectorIds\":[],\"side\":\"TOP\"},\"type\":\"ConnectorPlacement.EquallySpacedRectSide\",\"uuid\":\"a860ecae-5cde-45ef-a487-fdb4fb7390aa\"},{\"content\":{\"connectorIds\":[\"In3\"],\"side\":\"BOTTOM\"},\"type\":\"ConnectorPlacement.EquallySpacedRectSide\",\"uuid\":\"925435f5-0fb8-4a67-9f76-fe99b5b92634\"},{\"content\":{\"connectorIds\":[],\"side\":\"HIDDEN\"},\"type\":\"ConnectorPlacement.EquallySpacedRectSide\",\"uuid\":\"e6f3edac-a41a-4276-8ae6-cd8be9b02af9\"}]},\"type\":\"ConnectorPlacement.EquallySpacedConnector\",\"uuid\":\"0e32a9d0-da82-46c8-ab50-9de41c4380a9\"}],\"packageUris\":[\"http://schema.mathworks.com/mf0/Connector/R2020b\"],\"version\":\"1.0\"}"
  weight_register : Subsystem
  Valid : Outport
  Out1 : Outport  Port=2
  Out2 : Outport  Port=3
  Out3 : Outport  Port=4
  Out4 : Outport  Port=5
  Out5 : Outport  Port=6
  Out6 : Outport  Port=7
  Out7 : Outport  Port=8
  Out8 : Outport  Port=9
  Out9 : Outport  Port=10
  Out10 : Outport  Port=11
  Out11 : Outport  Port=12
  Out12 : Outport  Port=13
  Out13 : Outport  Port=14
  Out14 : Outport  Port=15
  Out15 : Outport  Port=16
  Out16 : Outport  Port=17
  Out17 : Outport  Port=18
  Out18 : Outport  Port=19
  wires:
  weight_register/4(Out5) -> Out4/1
  LIne Buffer/2(valid) -> Window Selector/2(valid)
  Window Selector/8(Out8) -> Out17/1
  weight_register/6(Out7) -> Out6/1
  weight_data/1 -> Delay4/1
  weight_register/9(Out1) -> Out9/1
  weight_data_valid/1 -> Delay5/1
  weight_register/2(Out3) -> Out2/1
  stride/1 -> Window Selector/3(stride)
  Feature_Height/1 -> LIne Buffer/6(Feature_Height)
  Delay4/1 -> weight_register/1(In1)
  LIne Buffer/1(pixel) -> Window Selector/1(In1)
  Stream_In/1 -> LIne Buffer/1(Stream_In)
  Delay5/1 -> weight_register/Enable
  Weight_Width/1 -> LIne Buffer/3(Weight_Width)
  weight_register/5(Out6) -> Out5/1
  weight_register/1(Out2) -> Out1/1
  Window Selector/4(Out4) -> Out13/1
  Feature_Width/1 -> LIne Buffer/5(Feature_Width)
  Window Selector/2(Out2) -> Out11/1
  weight_register/3(Out4) -> Out3/1
  Feature_Area/1 -> LIne Buffer/4(Feature_Area)
  Stream_Valid/1 -> LIne Buffer/2(Stream_Valid)
  weight_register/8(Out9) -> Out8/1
  weight_register/7(Out8) -> Out7/1
  Window Selector/5(Out5) -> Out14/1
  Window Selector/3(Out3) -> Out12/1
  Window Selector/9(Out9) -> Out18/1
  Window Selector/6(Out6) -> Out15/1
  Window Selector/7(Out7) -> Out16/1
  Window Selector/1(Out1) -> Out10/1
  Window Selector/10(Valid) -> Valid/1

== system PE_V2_0/2DConvPE1 V2.0/MaxPooling ==
  Stream_Valid : Inport
  Stream_In : Inport  Port=2
  ByPass : Inport  Port=3
  stride : Inport  Port=4
  Window_Width : Inport  Port=5
  Feature_Area : Inport  Port=6
  Feature_Width : Inport  Port=7
  Feature_Height : Inport  Port=8
  Comparator : Subsystem
  Constant : Constant  Value=0  OutDataTypeStr=int32
  Delay{,1..6,36} (8 alike) : Delay  DelayLength=1
  Line Buffer1 : Subsystem
  OutValidGen : Subsystem
  Switch : Switch  Criteria=u2 > Threshold
  Switch1 : Switch  Criteria=u2 > Threshold
  Terminator1 : Terminator
  dataSwitch : Switch  Criteria=u2 > Threshold
  validSwitch : Switch  Criteria=u2 > Threshold
  window Selector : Subsystem
  outdata : Outport
  Valid : Outport  Port=2
  wires:
  window Selector/3(Out3) -> Delay3/1
  OutValidGen/1(Out1) -> window Selector/2(valid)
  Feature_Width/1 -> Line Buffer1/4(Feature_Width)
  Line Buffer1/3(shftEnable) -> Terminator1/1
  Window_Width/1 -> OutValidGen/2(Window_Width)
  window Selector/5(Valid) -> Delay5/1
  window Selector/1(Out1) -> Delay/1
  Line Buffer1/1(pixel) -> Delay2/1
  Line Buffer1/2(ctrl) -> OutValidGen/1(ctrl)
  window Selector/2(Out2) -> Delay6/1
  window Selector/4(Out4) -> Delay4/1
  Feature_Area/1 -> Line Buffer1/3(Feature_Area)
  Feature_Height/1 -> OutValidGen/3(Feature_Height)
  stride/1 -> window Selector/3(step)
  Delay1/1 -> validSwitch/1, Switch1/3
  Comparator/1(Out1) -> dataSwitch/3
  Delay36/1 -> dataSwitch/1, Switch/3
  ByPass/1 -> validSwitch/2, dataSwitch/2, Switch1/2, Switch/2
  dataSwitch/1 -> outdata/1
  validSwitch/1 -> Valid/1
  Constant/1 -> Switch1/1, Switch/1
  Switch/1 -> Line Buffer1/1(Stream_In)
  Switch1/1 -> Line Buffer1/2(Stream_Valid)
  Comparator/2(outvalid) -> validSwitch/3
  Stream_In/1 -> Delay36/1
  Stream_Valid/1 -> Delay1/1
  Delay2/1 -> window Selector/1(pixel)
  Delay/1 -> Comparator/1(In1)
  Delay5/1 -> Comparator/5(Valid)
  Delay4/1 -> Comparator/4(In4)
  Delay3/1 -> Comparator/3(In3)
  Delay6/1 -> Comparator/2(In2)

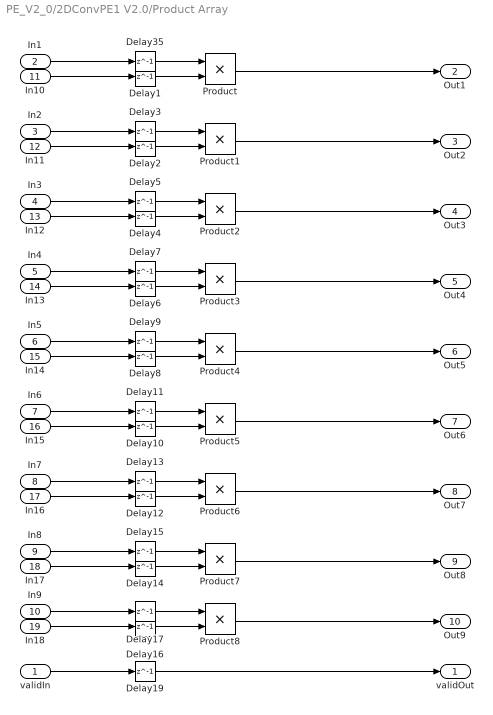
== system PE_V2_0/2DConvPE1 V2.0/Product Array ==
  validIn : Inport
  In1 : Inport  Port=2
  In2 : Inport  Port=3
  In3 : Inport  Port=4
  In4 : Inport  Port=5
  In5 : Inport  Port=6
  In6 : Inport  Port=7
  In7 : Inport  Port=8
  In8 : Inport  Port=9
  In9 : Inport  Port=10
  In10 : Inport  Port=11
  In11 : Inport  Port=12
  In12 : Inport  Port=13
  In13 : Inport  Port=14
  In14 : Inport  Port=15
  In15 : Inport  Port=16
  In16 : Inport  Port=17
  In17 : Inport  Port=18
  In18 : Inport  Port=19
  Delay{1..17,19,35} (19 alike) : Delay  DelayLength=1
  Product{,1..8} (9 alike) : Product
  validOut : Outport
  Out1 : Outport  Port=2
  Out2 : Outport  Port=3
  Out3 : Outport  Port=4
  Out4 : Outport  Port=5
  Out5 : Outport  Port=6
  Out6 : Outport  Port=7
  Out7 : Outport  Port=8
  Out8 : Outport  Port=9
  Out9 : Outport  Port=10
  wires:
  Product/1 -> Out1/1
  In4/1 -> Delay7/1
  Product4/1 -> Out5/1
  In8/1 -> Delay15/1
  In17/1 -> Delay14/1
  In9/1 -> Delay17/1
  In12/1 -> Delay4/1
  In7/1 -> Delay13/1
  In1/1 -> Delay35/1
  In13/1 -> Delay6/1
  Product1/1 -> Out2/1
  In16/1 -> Delay12/1
  In10/1 -> Delay1/1
  In14/1 -> Delay8/1
  In18/1 -> Delay16/1
  Product8/1 -> Out9/1
  Product7/1 -> Out8/1
  In6/1 -> Delay11/1
  In2/1 -> Delay3/1
  In11/1 -> Delay2/1
  In15/1 -> Delay10/1
  In5/1 -> Delay9/1
  In3/1 -> Delay5/1
  Product3/1 -> Out4/1
  Product2/1 -> Out3/1
  Product5/1 -> Out6/1
  Product6/1 -> Out7/1
  validIn/1 -> Delay19/1
  Delay1/1 -> Product/2
  Delay35/1 -> Product/1
  Delay3/1 -> Product1/1
  Delay2/1 -> Product1/2
  Delay5/1 -> Product2/1
  Delay4/1 -> Product2/2
  Delay7/1 -> Product3/1
  Delay6/1 -> Product3/2
  Delay8/1 -> Product4/2
  Delay9/1 -> Product4/1
  Delay11/1 -> Product5/1
  Delay10/1 -> Product5/2
  Delay13/1 -> Product6/1
  Delay12/1 -> Product6/2
  Delay14/1 -> Product7/2
  Delay15/1 -> Product7/1
  Delay17/1 -> Product8/1
  Delay16/1 -> Product8/2
  Delay19/1 -> validOut/1

== system PE_V2_0/2DConvPE1 V2.0/ReLU ==
  validIn : Inport
  data_in : Inport  Port=2
  byPass : Inport  Port=3
  Compare To Zero : simulink/Logic and Bit Operations/Compare To Zero  relop=>  OutDataTypeStr=boolean
  Constant : Constant  Value=0  OutDataTypeStr=int32
  Delay1 : Delay  DelayLength=1
  Delay36 : Delay  DelayLength=1
  Switch : Switch  Criteria=u2 > Threshold
  Switch1 : Switch  Criteria=u2 > Threshold
  valildOut : Outport
  data_ReLU : Outport  Port=2
  wires:
  Constant/1 -> Switch/3
  Delay36/1 -> Switch1/1, Switch/1, Compare To Zero/1
  Compare To Zero/1 -> Switch/2
  Switch/1 -> Switch1/3
  byPass/1 -> Switch1/2
  Switch1/1 -> data_ReLU/1
  Delay1/1 -> valildOut/1
  data_in/1 -> Delay36/1
  validIn/1 -> Delay1/1

== system PE_V2_0/2DConvPE1 V2.0/Subsystem ==
  In1 : Inport
  Bus Selector : BusSelector  OutputSignals=signal1,signal2
  pool_step : Outport
  pool_Width : Outport  Port=2
  wires:
  Bus Selector/2 -> pool_Width/1  "<signal2>"
  Bus Selector/1 -> pool_step/1  "<signal1>"
  In1/1 -> Bus Selector/1
